simulink model "vehstlin_mdl"  (Simulink 8.8)
settings: Solver=VariableStepAuto  StartTime=0.0  StopTime=10.0  RelTol=1e-3
values from neighbouring files (symbols this model uses):
  A = [a11, 0, a13, 0 ... (first row only)    [vehstlin_sseval.m]
  B = [b11 ... (first row only)    [vehstlin_sseval.m]
  C = [0, 0, 1, 0]    [vehstlin_sseval.m]
  D = 0    [vehstlin_sseval.m]
  v = 20    [vehstlin_param.m]
libraries: simulink x1
settings Model: Creator=hfe2bp  LastModifiedBy=hfe2bp
settings DataIOCC: LimitDataPoints=off  SaveFormat=Dataset  SignalLoggingSaveFormat=Dataset
settings OptimizationCC: LifeSpan=auto
settings DebuggingCC: UnderspecifiedInitializationDetection=Simplified  MergeDetectMultiDrivingBlocksExec=error  FcnCallInpInsideContextMsg=error  StateNameClashWarn=none  SFUnexpectedBacktrackingDiag=error  SFNoUnconditionalDefaultTransitionDiag=error  SFExecutionAtInitializationDiag=warning
settings HardwareCC: ProdBitPerPointer=64  ProdBitPerSizeT=64  ProdBitPerPtrDiffT=64  ProdLargestAtomicFloat=Float  ProdIntDivRoundTo=Zero  ProdEndianess=LittleEndian  ProdWordSize=64  ProdHWDeviceType=Intel->x86-64 (Windows64)
settings ModelReferenceCC: PropagateSignalLabelsOutOfModel=on
settings GRTTargetCC: TargetLangStandard=C99 (ISO)  GeneratePreprocessorConditionals=Use local settings  CombineOutputUpdateFcns=on  GRTInterface=off
settings ConfigComp: CovMetricSettings=dwe  CovHtmlReporting=off  CovSaveCumulativeToWorkspaceVar=off  CovSaveSingleToWorkspaceVar=off  CovExternalEMLEnable=on

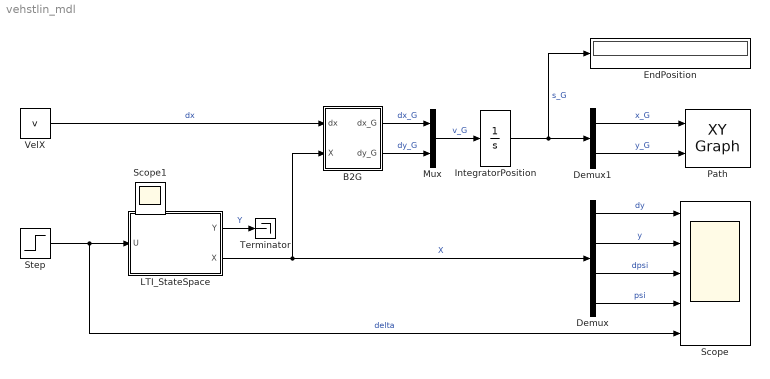
== system vehstlin_mdl ==
  B2G : Subsystem
  Demux : Demux
  Demux1 : Demux  Outputs=2
  EndPosition : Display
  IntegratorPosition : Integrator
  LTI_StateSpace : Subsystem
  Mux : Mux  Inputs=2
  Path : simulink/Sinks/XY Graph  xmin=0  xmax=300  ymin=0  ymax=200  st=-1
  Scope : Scope  NumInputPorts=5
  Step : Step  After=1/180*pi  SampleTime=0
  Terminator : Terminator
  VelX : Constant  Value=v
  Scope1 : Scope
  wires:
  Step/1 -> LTI_StateSpace/1(U), Scope/5  "delta"
  LTI_StateSpace/1(Y) -> Terminator/1  "Y"
  Demux/1 -> Scope/1  "dy"
  Demux/2 -> Scope/2  "y"
  Demux/3 -> Scope/3  "dpsi"
  Demux/4 -> Scope/4  "psi"
  VelX/1 -> B2G/1(dx)  "dx"
  B2G/1(dx_G) -> Mux/1  "dx_G"
  B2G/2(dy_G) -> Mux/2  "dy_G"
  Mux/1 -> IntegratorPosition/1  "v_G"
  IntegratorPosition/1 -> EndPosition/1, Demux1/1  "s_G"
  Demux1/1 -> Path/1  "x_G"
  Demux1/2 -> Path/2  "y_G"
  LTI_StateSpace/2(X) -> Demux/1, B2G/2(X)  "X"

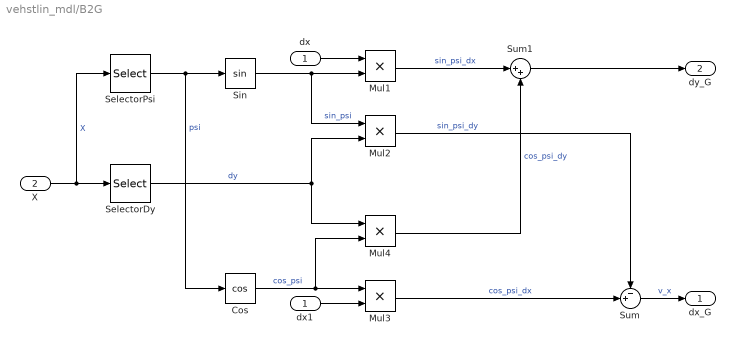
== system vehstlin_mdl/B2G ==
  dx : Inport
  X : Inport  Port=2
  Cos : Trigonometry  Operator=cos
  Mul{1..4} (4 alike) : Product  Inputs=**
  SelectorDy : Selector  InputPortWidth=4  IndexOptions=Index vector (dialog)  Indices=[1]  OutputSizes=1
  SelectorPsi : Selector  InputPortWidth=4  IndexOptions=Index vector (dialog)  Indices=[4]  OutputSizes=1
  Sin : Trigonometry
  Sum : Sum  Inputs=-+|
  Sum1 : Sum  Inputs=|++
  dx1 : InportShadow
  dx_G : Outport
  dy_G : Outport  Port=2
  wires:
  Cos/1 -> Mul4/2, Mul3/1  "cos_psi"
  Sin/1 -> Mul2/1, Mul1/2  "sin_psi"
  SelectorPsi/1 -> Cos/1, Sin/1  "psi"
  X/1 -> SelectorPsi/1, SelectorDy/1  "X"
  SelectorDy/1 -> Mul4/1, Mul2/2  "dy"
  dx/1 -> Mul1/1
  dx1/1 -> Mul3/2
  Mul1/1 -> Sum1/1  "sin_psi_dx"
  Mul2/1 -> Sum/1  "sin_psi_dy"
  Mul4/1 -> Sum1/2  "cos_psi_dy"
  Mul3/1 -> Sum/2  "cos_psi_dx"
  Sum/1 -> dx_G/1  "v_x"
  Sum1/1 -> dy_G/1

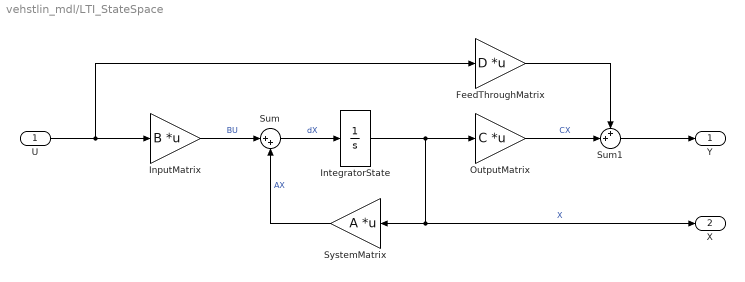
== system vehstlin_mdl/LTI_StateSpace ==
  U : Inport
  FeedThroughMatrix : Gain  Gain=D  Multiplication=Matrix(K*u)
  InputMatrix : Gain  Gain=B  Multiplication=Matrix(K*u)
  IntegratorState : Integrator
  OutputMatrix : Gain  Gain=C  Multiplication=Matrix(K*u)
  Sum : Sum  Inputs=|++
  Sum1 : Sum  Inputs=++|
  SystemMatrix : Gain  Gain=A  Multiplication=Matrix(K*u)
  Y : Outport
  X : Outport  Port=2
  wires:
  Sum/1 -> IntegratorState/1  "dX"
  IntegratorState/1 -> X/1, SystemMatrix/1, OutputMatrix/1  "X"
  SystemMatrix/1 -> Sum/2  "AX"
  InputMatrix/1 -> Sum/1  "BU"
  U/1 -> InputMatrix/1, FeedThroughMatrix/1
  OutputMatrix/1 -> Sum1/2  "CX"
  Sum1/1 -> Y/1
  FeedThroughMatrix/1 -> Sum1/1
